simulink model "linear_sys_simple"  (R2021b)
settings: Solver=ode4  StartTime=0  StopTime=T_end  FixedStep=dt  RelTol=1e-3
values from neighbouring files (symbols this model uses):
  delay_board_y = delay_board_x    (= 0.01)    [data.m]
  dt = 1e-3    (= 0.001)    [data.m]
  g = 9.81    [data.m]
  IC = [0.0 0.0]    [data.m]    (also in postproc2.m)
  Kbbx = (mb * g * rb^2 * rm) / ((mb * rb^2 + Jb) * Ly)    (= 0.952057453416)    [data.m]
  Kbby = (mb * g * rb^2 * rm) / ((mb * rb^2 + Jb) * Lx)    (= 1.22502497502)    [data.m]
  PID_sim = PID(9)    [data.m]    (also in postproc2.m = PID(PID_idx(ii)))
  rate_limit = 20    [data.m]
  rf_amp = 1    [data.m]
  rf_treshold = 2    [data.m]
  tau_mot_y = tau_mot_x    (= 0.029)    [data.m]
  tau_sens_y = tau_sens_x    (= 0.079)    [data.m]
  V2theta_y = V2theta_x    (= 0.222)    [data.m]
undefined symbols (not defined in the file or in its folder): ref
libraries: simulink x4, slpidlib x2
settings Model: Creator=Daniele Oranges  LastModifiedBy=Daniele Oranges
settings DataIOCC: SaveFormat=StructureWithTime
settings OptimizationCC: BlockReduction=off  BufferReuse=off
settings DebuggingCC: AlgebraicLoopMsg=none  UnconnectedInputMsg=none  UnconnectedOutputMsg=none  UnconnectedLineMsg=none
settings ExplorerConfigSet: SimMechanicsOpenEditorOnUpdate=off

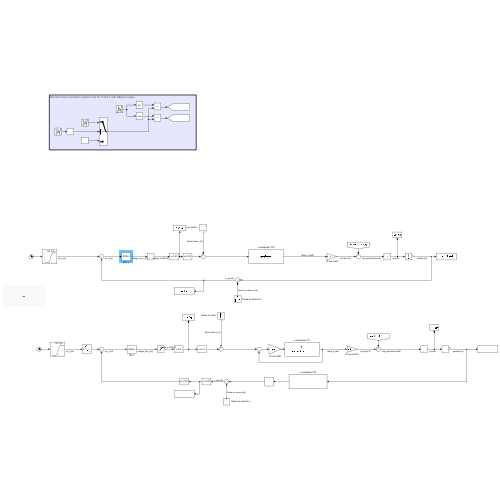
[thumbnail: Simulink's stored preview of the top-level diagram]
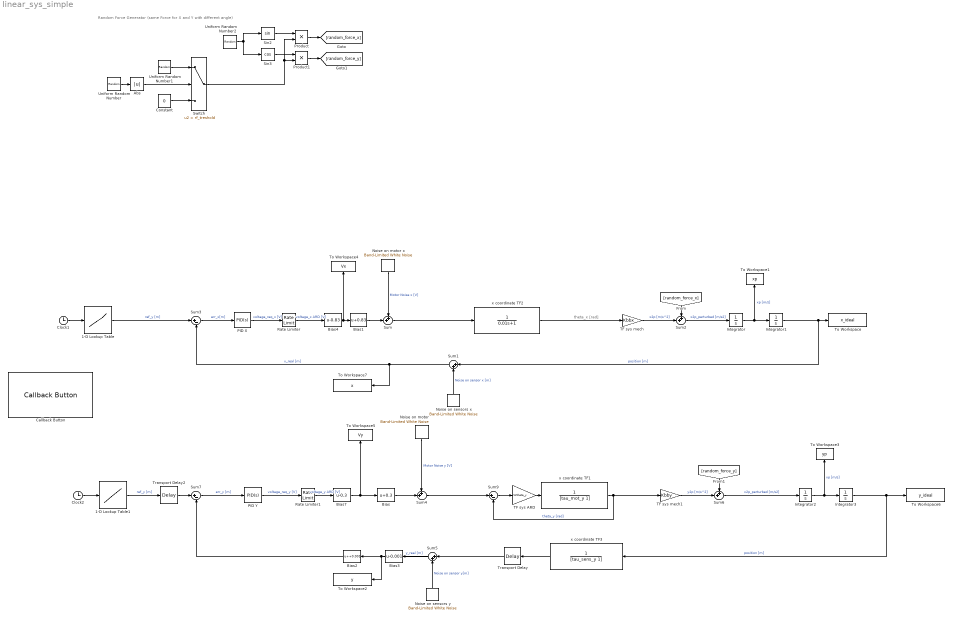
== system linear_sys_simple ==
  note: theta_x [rad]
  note: Random Force Generator (same Force for X and Y with different angle)
  1-D Lookup Table : Lookup_n-D  NumberOfTableDimensions=1  BreakpointsForDimension1=ref.x.t  Table=ref.x.v  InternalRulePriority=Speed  RndMeth=Simplest  InputSameDT=on
  1-D Lookup Table1 : Lookup_n-D  NumberOfTableDimensions=1  BreakpointsForDimension1=ref.y.t  Table=ref.y.v  InternalRulePriority=Speed  RndMeth=Simplest  InputSameDT=on
  Abs : Abs
  Bias : Bias  Bias=0.3
  Bias1 : Bias  Bias=0.83
  Bias2 : Bias  Bias=+0.001
  Bias3 : Bias  Bias=-0.001
  Bias4 : Bias  Bias=-0.83
  Bias7 : Bias  Bias=-0.3
  Callback Button : CallbackButton  ButtonText=Initialize Data
      settings: ClickFcn=|
      | clear
      | data
  Clock1 : Clock
  Clock2 : Clock
  Constant : Constant  Value=0
  Integrator : Integrator
  Integrator1 : Integrator  InitialCondition=IC(1)
  Integrator2 : Integrator
  Integrator3 : Integrator  InitialCondition=IC(1)
  Noise on motor : simulink/Sources/Band-Limited White Noise  Cov=2e-4  Ts=dt  seed=[23341]
  Noise on motor x : simulink/Sources/Band-Limited White Noise  Cov=2e-4  Ts=dt  seed=[23341]
  Noise on sensors x : simulink/Sources/Band-Limited White Noise  Cov=Nsensor  Ts=dt  seed=[23341]
  Noise on sensors y : simulink/Sources/Band-Limited White Noise  Cov=Nsensor  Ts=dt  seed=[23341]
  PID X : slpidlib/PID Controller  Controller=PID  Form=Parallel  TimeDomain=Continuous-time  UseExternalTs=off  SampleTime=-1  IntegratorMethod=Forward Euler  FilterMethod=Forward Euler  ControllerParametersSource=internal  P=1.00004447296947  I=0.0148165576450285  D=14.9972725515647  UseFilter=on  N=290.233629519559  TunerSelectOption=Transfer Function Based (PID Tuner App)  InitialConditionSource=internal  InitialConditionForIntegrator=0  InitialConditionForFilter=0  DifferentiatorICPrevScaledInput=0  ExternalReset=none  TrackingMode=off  Kt=1  LimitOutput=off  SatLimitsSource=internal  UpperSaturationLimit=inf  LowerSaturationLimit=-inf  LinearizeAsGain=on  AntiWindupMode=none  Kb=1  POutMin=[]  POutMax=[]  IOutMin=[]  IOutMax=[]  DOutMin=[]  DOutMax=[]  NOutMin=[]  NOutMax=[]  SumOutMin=[]  SumOutMax=[]  SaturationOutMin=[]  SaturationOutMax=[]  PParamMin=[]  PParamMax=[]  IParamMin=[]  IParamMax=[]  DParamMin=[]  DParamMax=[]  NParamMin=[]  NParamMax=[]  KbParamMin=[]  KbParamMax=[]  KtParamMin=[]  KtParamMax=[]  KbOutMin=[]  KbOutMax=[]  KtOutMin=[]  KtOutMax=[]  IntegratorOutMin=[]  IntegratorOutMax=[]  FilterOutMin=[]  FilterOutMax=[]  SumI1OutMin=[]  SumI1OutMax=[]  SumI2OutMin=[]  SumI2OutMax=[]  SumI3OutMin=[]  SumI3OutMax=[]  SumI4OutMin=[]  SumI4OutMax=[]  SumDOutMin=[]  SumDOutMax=[]  DifferentiatorOutMin=[]  DifferentiatorOutMax=[]  FilterDiffOutCoefMin=[]  FilterDiffOutCoefMax=[]  ReciprocalOutMin=[]  ReciprocalOutMax=[]  SumDenOutMin=[]  SumDenOutMax=[]  SumNumOutMin=[]  SumNumOutMax=[]  DivideOutMin=[]  DivideOutMax=[]  UdiffTsProdOutMin=[]  UdiffTsProdOutMax=[]  NTsProdOutMin=[]  NTsProdOutMax=[]  UintegralTsProdOutMin=[]  UintegralTsProdOutMax=[]  UngainTsProdOutMin=[]  UngainTsProdOutMax=[]  IntegratorContinuousStateAttributes=''  IntegratorStateMustResolveToSignalObject=off  IntegratorRTWStateStorageClass=Auto  FilterContinuousStateAttributes=''  FilterStateMustResolveToSignalObject=off  FilterRTWStateStorageClass=Auto  ParallelPVariant=InternalParameters  IdealPVariant=Disabled  IVariant=InternalParameters  DVariant=InternalParameters  IntegratorVariant=Continuous  SatVariant=Disabled  AWVariant=Passthrough  PCopyVariant=Disabled  TRVariant=Disabled  FdbkBlocksVariant=Forward  IdealPFdbkVariant=Disabled  SatFdbkVariant=Disabled  DerivativeFilterVariant=ContFilter  NVariant=InternalParameters  NCopyVariant=Disabled  FilterICVariant=InternalICsFilter  IntegratorICVariant=InternalICs  ExternalResetVariant=Disabled  TRSumVariant=Passthrough  SumFdbkVariant=Disabled  SumVariant=Sum_PID  TsampFilterVariant=InternalTs  TsampNgainVariant=Passthrough  TsampIntegralVariant=Passthrough  ExternalSaturationOutDataTypeStr=Inherit: Same as second input
  PID Y : slpidlib/PID Controller  Controller=PID  Form=Parallel  TimeDomain=Continuous-time  UseExternalTs=off  SampleTime=-1  IntegratorMethod=Forward Euler  FilterMethod=Forward Euler  ControllerParametersSource=internal  P=PID_sim.Kp  I=PID_sim.Ki  D=PID_sim.Kd  UseFilter=on  N=PID_sim.filter  TunerSelectOption=Transfer Function Based (PID Tuner App)  InitialConditionSource=internal  InitialConditionForIntegrator=0  InitialConditionForFilter=0  DifferentiatorICPrevScaledInput=0  ExternalReset=none  TrackingMode=off  Kt=1  LimitOutput=off  SatLimitsSource=internal  UpperSaturationLimit=inf  LowerSaturationLimit=-inf  LinearizeAsGain=on  AntiWindupMode=none  Kb=1  POutMin=[]  POutMax=[]  IOutMin=[]  IOutMax=[]  DOutMin=[]  DOutMax=[]  NOutMin=[]  NOutMax=[]  SumOutMin=[]  SumOutMax=[]  SaturationOutMin=[]  SaturationOutMax=[]  PParamMin=[]  PParamMax=[]  IParamMin=[]  IParamMax=[]  DParamMin=[]  DParamMax=[]  NParamMin=[]  NParamMax=[]  KbParamMin=[]  KbParamMax=[]  KtParamMin=[]  KtParamMax=[]  KbOutMin=[]  KbOutMax=[]  KtOutMin=[]  KtOutMax=[]  IntegratorOutMin=[]  IntegratorOutMax=[]  FilterOutMin=[]  FilterOutMax=[]  SumI1OutMin=[]  SumI1OutMax=[]  SumI2OutMin=[]  SumI2OutMax=[]  SumI3OutMin=[]  SumI3OutMax=[]  SumI4OutMin=[]  SumI4OutMax=[]  SumDOutMin=[]  SumDOutMax=[]  DifferentiatorOutMin=[]  DifferentiatorOutMax=[]  FilterDiffOutCoefMin=[]  FilterDiffOutCoefMax=[]  ReciprocalOutMin=[]  ReciprocalOutMax=[]  SumDenOutMin=[]  SumDenOutMax=[]  SumNumOutMin=[]  SumNumOutMax=[]  DivideOutMin=[]  DivideOutMax=[]  UdiffTsProdOutMin=[]  UdiffTsProdOutMax=[]  NTsProdOutMin=[]  NTsProdOutMax=[]  UintegralTsProdOutMin=[]  UintegralTsProdOutMax=[]  UngainTsProdOutMin=[]  UngainTsProdOutMax=[]  IntegratorContinuousStateAttributes=''  IntegratorStateMustResolveToSignalObject=off  IntegratorRTWStateStorageClass=Auto  FilterContinuousStateAttributes=''  FilterStateMustResolveToSignalObject=off  FilterRTWStateStorageClass=Auto  ParallelPVariant=InternalParameters  IdealPVariant=Disabled  IVariant=InternalParameters  DVariant=InternalParameters  IntegratorVariant=Continuous  SatVariant=Disabled  AWVariant=Passthrough  PCopyVariant=Disabled  TRVariant=Disabled  FdbkBlocksVariant=Forward  IdealPFdbkVariant=Disabled  SatFdbkVariant=Disabled  DerivativeFilterVariant=ContFilter  NVariant=InternalParameters  NCopyVariant=Disabled  FilterICVariant=InternalICsFilter  IntegratorICVariant=InternalICs  ExternalResetVariant=Disabled  TRSumVariant=Passthrough  SumFdbkVariant=Disabled  SumVariant=Sum_PID  TsampFilterVariant=InternalTs  TsampNgainVariant=Passthrough  TsampIntegralVariant=Passthrough  ExternalSaturationOutDataTypeStr=Inherit: Same as second input
  Product : Product
  Product1 : Product
  Rate Limiter : RateLimiter  RisingSlewLimit=rate_limit  FallingSlewLimit=-rate_limit  SampleTimeMode=inherited
  Rate Limiter1 : RateLimiter  RisingSlewLimit=rate_limit  FallingSlewLimit=-rate_limit  SampleTimeMode=inherited
  Sin2 : Trigonometry
  Sin3 : Trigonometry  Operator=cos
  Sum{,2,4,6} (4 alike) : Sum  Inputs=++|
  Sum1 : Sum  Inputs=|++
  Sum3 : Sum  Inputs=|+-
  Sum5 : Sum  Inputs=|++
  Sum7 : Sum  Inputs=|+-
  Sum9 : Sum  Inputs=|+-
  Switch : Switch  Criteria=u2 > Threshold  Threshold=rf_treshold
  TF sys ARD : Gain  Gain=V2theta_y
  TF sys mech : Gain  Gain=Kbbx
  TF sys mech1 : Gain  Gain=Kbby
  To Workspace : ToWorkspace  VariableName=x_ideal  SaveFormat=Timeseries  SampleTime=-1
  To Workspace1 : ToWorkspace  VariableName=xp  SaveFormat=Timeseries  SampleTime=-1
  To Workspace2 : ToWorkspace  VariableName=y  SaveFormat=Timeseries  SampleTime=-1
  To Workspace3 : ToWorkspace  VariableName=yp  SaveFormat=Timeseries  SampleTime=-1
  To Workspace4 : ToWorkspace  VariableName=Vx  SaveFormat=Timeseries  SampleTime=-1
  To Workspace5 : ToWorkspace  VariableName=Vy  SaveFormat=Timeseries  SampleTime=-1
  To Workspace6 : ToWorkspace  VariableName=y_ideal  SaveFormat=Timeseries  SampleTime=-1
  To Workspace7 : ToWorkspace  VariableName=x  SaveFormat=Timeseries  SampleTime=-1
  Transport Delay : TransportDelay  DelayTime=delay_board_y
  Transport Delay2 : TransportDelay  DelayTime=dt
  Uniform Random Number : UniformRandomNumber  SampleTime=round(rand(1)*10)
  Uniform Random Number1 : UniformRandomNumber  Minimum=-rf_amp/g  Maximum=rf_amp/g  SampleTime=100*dt
  Uniform Random Number2 : UniformRandomNumber  Minimum=0  Maximum=2*pi  SampleTime=round(rand(1)*10)
  x coordinate TF1 : TransferFcn  Denominator=[tau_mot_y 1]
  x coordinate TF2 : TransferFcn  Denominator=[0.01 1]
  x coordinate TF3 : TransferFcn  Denominator=[tau_sens_y 1]
  wires:
  Integrator/1 -> Integrator1/1, To Workspace1/1  "xp [m/s]"
  Noise on sensors x/1 -> Sum1/2  "Noise on sensor x [m]"
  Integrator1/1 -> Sum1/1, To Workspace/1  "position [m]"
  x coordinate TF2/1 -> TF sys mech/1
  Noise on motor x/1 -> Sum/1  "Motor Noise x [V]"
  TF sys mech/1 -> Sum2/2  "x2p [m/s^2]"
  TF sys mech1/1 -> Sum6/2  "y2p [m/s^2]"
  Noise on motor/1 -> Sum4/1  "Motor Noise y [V]"
  PID Y/1 -> Rate Limiter1/1  "voltage_req_y [V]"
  Sum7/1 -> PID Y/1  "err_y [m]"
  Noise on sensors y/1 -> Sum5/2  "Noise on sensor y[m]"
  Sum5/1 -> Bias3/1  "y_real [m]"
  Clock1/1 -> 1-D Lookup Table/1
  Clock2/1 -> 1-D Lookup Table1/1
  Sum1/1 -> Sum3/2, To Workspace7/1  "x_real [m]"
  Sum2/1 -> Integrator/1  "x2p_perturbed [m/s2]"
  Rate Limiter/1 -> Bias4/1  "voltage_x ARD [V]"
  Uniform Random Number1/1 -> Switch/1
  Uniform Random Number/1 -> Abs/1
  Constant/1 -> Switch/3
  Switch/1 -> Product1/2, Product/2
  Product/1 -> [random_force_x]
  Abs/1 -> Switch/2
  [random_force_x] -> Sum2/1
  Uniform Random Number2/1 -> Sin3/1, Sin2/1
  Sin2/1 -> Product/1
  Sin3/1 -> Product1/1
  Product1/1 -> [random_force_y]
  [random_force_y] -> Sum6/1
  Rate Limiter1/1 -> Bias7/1  "voltage_y ARD [V]"
  Bias/1 -> Sum4/2
  1-D Lookup Table1/1 -> Transport Delay2/1  "ref_y [m]"
  Transport Delay2/1 -> Sum7/1
  Bias1/1 -> Sum/2
  Sum/1 -> x coordinate TF2/1
  Sum9/1 -> TF sys ARD/1
  x coordinate TF1/1 -> TF sys mech1/1, Sum9/2  "theta_y [rad]"
  TF sys ARD/1 -> x coordinate TF1/1
  x coordinate TF3/1 -> Transport Delay/1
  Transport Delay/1 -> Sum5/1
  Sum4/1 -> Sum9/1
  Integrator2/1 -> Integrator3/1, To Workspace3/1  "xp [m/s]"
  Integrator3/1 -> To Workspace6/1, x coordinate TF3/1  "position [m]"
  Sum6/1 -> Integrator2/1  "x2p_perturbed [m/s2]"
  1-D Lookup Table/1 -> Sum3/1  "ref_y [m]"
  Bias2/1 -> Sum7/2
  Bias3/1 -> Bias2/1, To Workspace2/1
  Bias4/1 -> Bias1/1, To Workspace4/1
  Bias7/1 -> Bias/1, To Workspace5/1
  Sum3/1 -> PID X/1  "err_x[m]"
  PID X/1 -> Rate Limiter/1  "voltage_req_x [V]"
